simulink model "two"  (R2020b)
settings: Solver=VariableStepAuto  StartTime=0.0  StopTime=10.0  RelTol=1e-3
values from neighbouring files (symbols this model uses):
  be = 2.0    [variables.sldd]
  bv = 1.0    [variables.sldd]
  Ie = 1.0    [variables.sldd]
  Iv = 5.0    [variables.sldd]
  muk = 1.0    [variables.sldd]
  mus = 1.5    [variables.sldd]
  R = 1.0    [variables.sldd]
settings Model: Creator=USER  LastModifiedBy=USER

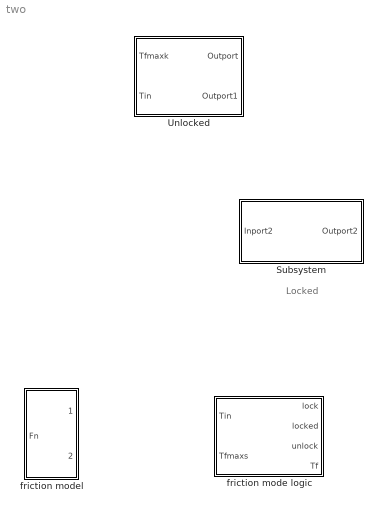
== system two ==
  note: Locked
  Subsystem : Subsystem
  Unlocked : Subsystem
  friction mode logic : Subsystem
  friction model : Subsystem

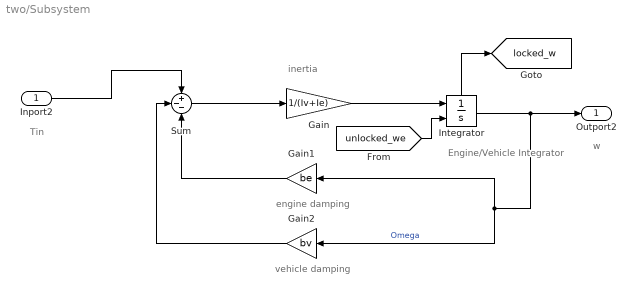
== system two/Subsystem ==
  note: w
  note: Tin
  note: inertia
  note: vehicle damping
  note: engine damping
  note: Engine/Vehicle
      | Integrator
  Inport2 : Inport
  Gain : Gain  Gain=1/(Iv+Ie)
  Gain1 : Gain  Gain=be
  Gain2 : Gain  Gain=bv
  Integrator : Integrator  InitialConditionSource=external  ShowStatePort=on
  Sum : Sum  Inputs=+--
  Outport2 : Outport
  tag scope: locked_w=global
  wires:
  [unlocked_we] -> Integrator/2
  Integrator/1 -> Outport2/1, Gain2/1, Gain1/1  "Omega"
  Gain/1 -> Integrator/1
  Integrator/State -> [locked_w]
  Sum/1 -> Gain/1
  Gain2/1 -> Sum/2
  Gain1/1 -> Sum/3
  Inport2/1 -> Sum/1

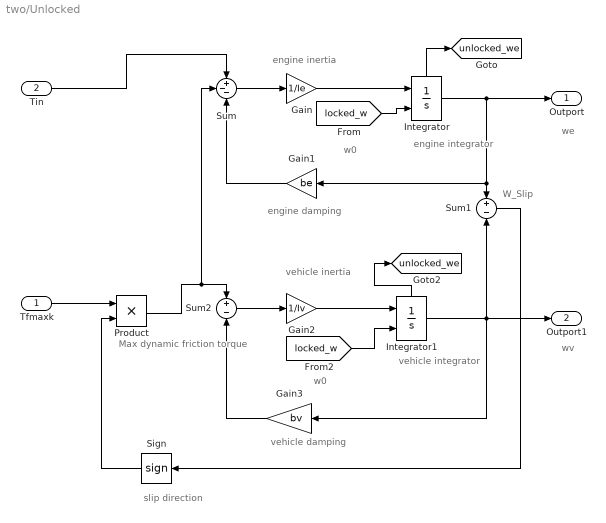
== system two/Unlocked ==
  note: we
  note: wv
  note: W_Slip
  note: vehicle
      | integrator
  note: engine
      | integrator
  note: w0
  note: w0
  note: engine damping
  note: engine inertia
  note: vehicle
      | inertia
  note: vehicle
      | damping
  note: slip direction
  note: Max
      | dynamic
      | friction
      | torque
  Tfmaxk : Inport
  Tin : Inport  Port=2
  Gain : Gain  Gain=1/Ie
  Gain1 : Gain  Gain=be
  Gain2 : Gain  Gain=1/Iv
  Gain3 : Gain  Gain=bv
  Integrator : Integrator  InitialConditionSource=external  ShowStatePort=on  ZeroCross=off
  Integrator1 : Integrator  InitialConditionSource=external  ShowStatePort=on  ZeroCross=off
  Product : Product
  Sign : Signum
  Sum : Sum  Inputs=+--
  Sum1 : Sum  Inputs=+-
  Sum2 : Sum  Inputs=+-
  Outport : Outport
  Outport1 : Outport  Port=2
  tag scope: unlocked_we=global
  wires:
  Sum/1 -> Gain/1
  Tfmaxk/1 -> Product/1
  Sum2/1 -> Gain2/1
  Sum1/1 -> Sign/1
  Integrator1/State -> [unlocked_we]
  Sign/1 -> Product/2
  Gain2/1 -> Integrator1/1
  Integrator/1 -> Outport/1, Gain1/1, Sum1/1
  [locked_w] -> Integrator1/2
  Integrator1/1 -> Outport1/1, Sum1/2, Gain3/1
  Product/1 -> Sum/2, Sum2/1
  Gain/1 -> Integrator/1
  Gain1/1 -> Sum/3
  Gain3/1 -> Sum2/2
  Tin/1 -> Sum/1
  [locked_w] -> Integrator/2
  Integrator/State -> [unlocked_we]

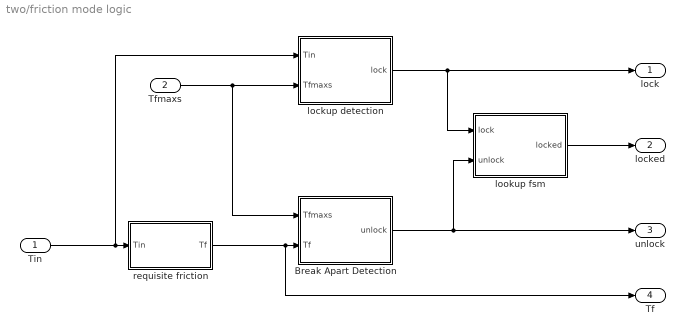
== system two/friction mode logic ==
  Tin : Inport
  Tfmaxs : Inport  Port=2
  Break Apart Detection : Subsystem
  lockup detection : Subsystem
  lookup fsm : Subsystem
  requisite friction : Subsystem
  lock : Outport
  locked : Outport  Port=2
  unlock : Outport  Port=3
  Tf : Outport  Port=4
  wires:
  Tfmaxs/1 -> Break Apart Detection/1(Tfmaxs), lockup detection/2(Tfmaxs)
  lockup detection/1(lock) -> lock/1, lookup fsm/1(lock)
  Break Apart Detection/1(unlock) -> unlock/1, lookup fsm/2(unlock)
  lookup fsm/1(locked) -> locked/1
  requisite friction/1(Tf) -> Tf/1, Break Apart Detection/2(Tf)
  Tin/1 -> lockup detection/1(Tin), requisite friction/1(Tin)

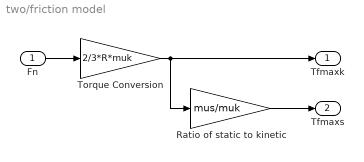
== system two/friction model ==
  Fn : Inport
  Ratio of static to kinetic : Gain  Gain=mus/muk  SaturateOnIntegerOverflow=on  OutDataTypeStr=Inherit: Same as input  ParamDataTypeStr=Inherit: Same as input
  Torque Conversion : Gain  Gain=2/3*R*muk  SaturateOnIntegerOverflow=on  OutDataTypeStr=Inherit: Same as input  ParamDataTypeStr=Inherit: Same as input
  Tfmaxk : Outport  InitialOutput=0  VectorParamsAs1DForOutWhenUnconnected=off
  Tfmaxs : Outport  Port=2  InitialOutput=0  VectorParamsAs1DForOutWhenUnconnected=off
  wires:
  Torque Conversion/1 -> Tfmaxk/1, Ratio of static to kinetic/1
  Fn/1 -> Torque Conversion/1
  Ratio of static to kinetic/1 -> Tfmaxs/1

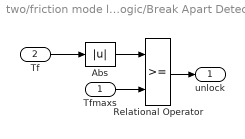
== system two/friction mode logic/Break Apart Detection ==
  Tfmaxs : Inport
  Tf : Inport  Port=2
  Abs : Abs  SaturateOnIntegerOverflow=on
  Relational Operator : RelationalOperator  OutDataTypeStr=boolean  RndMeth=Nearest  InputSameDT=on
  unlock : Outport  InitialOutput=0  VectorParamsAs1DForOutWhenUnconnected=off
  wires:
  Tf/1 -> Abs/1
  Relational Operator/1 -> unlock/1
  Abs/1 -> Relational Operator/1
  Tfmaxs/1 -> Relational Operator/2

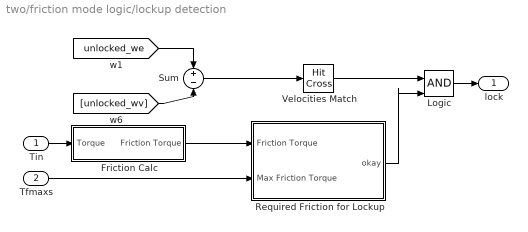
== system two/friction mode logic/lockup detection ==
  Tin : Inport
  Tfmaxs : Inport  Port=2
  Friction Calc : Subsystem
  Logic : Logic  IconShape=distinctive  OutDataTypeStr=boolean
  Required Friction for Lockup : Subsystem
  Sum : Sum  Inputs=+-  InputSameDT=on  SaturateOnIntegerOverflow=on  OutDataTypeStr=Inherit: Same as first input
  Velocities Match : HitCross
  lock : Outport  InitialOutput=0  VectorParamsAs1DForOutWhenUnconnected=off
  wires:
  Friction Calc/1(Friction Torque) -> Required Friction for Lockup/1(Friction Torque)
  Tfmaxs/1 -> Required Friction for Lockup/2(Max Friction Torque)
  Velocities Match/1 -> Logic/1
  Logic/1 -> lock/1
  Required Friction for Lockup/1(okay) -> Logic/2
  [unlocked_we] -> Sum/1
  [unlocked_wv] -> Sum/2
  Sum/1 -> Velocities Match/1
  Tin/1 -> Friction Calc/1(Torque)

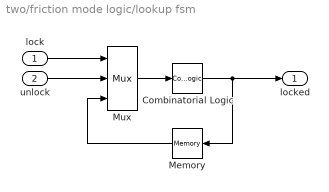
== system two/friction mode logic/lookup fsm ==
  lock : Inport
  unlock : Inport  Port=2
  Combinatorial Logic : CombinatorialLogic  TruthTable=[0;1;0;0;1;1;1;0]
  Memory : Memory
  Mux : Mux  Inputs=3
  locked : Outport  InitialOutput=0  VectorParamsAs1DForOutWhenUnconnected=off
  wires:
  Mux/1 -> Combinatorial Logic/1
  unlock/1 -> Mux/2
  Combinatorial Logic/1 -> locked/1, Memory/1
  lock/1 -> Mux/1
  Memory/1 -> Mux/3

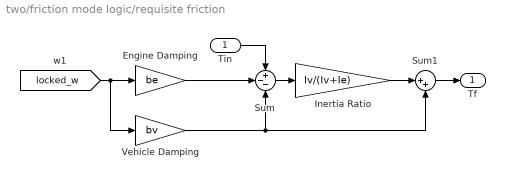
== system two/friction mode logic/requisite friction ==
  Tin : Inport
  Engine Damping : Gain  Gain=be  SaturateOnIntegerOverflow=on  OutDataTypeStr=Inherit: Same as input  ParamDataTypeStr=Inherit: Same as input
  Inertia Ratio : Gain  Gain=Iv/(Iv+Ie)  SaturateOnIntegerOverflow=on  OutDataTypeStr=Inherit: Same as input  ParamDataTypeStr=Inherit: Same as input
  Sum : Sum  Inputs=+--  InputSameDT=on  SaturateOnIntegerOverflow=on  OutDataTypeStr=Inherit: Same as first input
  Sum1 : Sum  Inputs=|++  InputSameDT=on  SaturateOnIntegerOverflow=on  OutDataTypeStr=Inherit: Same as first input
  Vehicle Damping : Gain  Gain=bv  SaturateOnIntegerOverflow=on  OutDataTypeStr=Inherit: Same as input  ParamDataTypeStr=Inherit: Same as input
  Tf : Outport  InitialOutput=0  VectorParamsAs1DForOutWhenUnconnected=off
  wires:
  [locked_w] -> Vehicle Damping/1, Engine Damping/1
  Engine Damping/1 -> Sum/2
  Vehicle Damping/1 -> Sum/3, Sum1/2
  Sum/1 -> Inertia Ratio/1
  Tin/1 -> Sum/1
  Inertia Ratio/1 -> Sum1/1
  Sum1/1 -> Tf/1

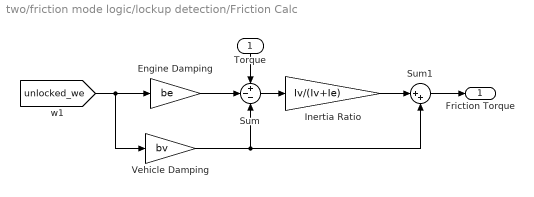
== system two/friction mode logic/lockup detection/Friction Calc ==
  Torque : Inport
  Engine Damping : Gain  Gain=be  SaturateOnIntegerOverflow=on  OutDataTypeStr=Inherit: Same as input  ParamDataTypeStr=Inherit: Same as input
  Inertia Ratio : Gain  Gain=Iv/(Iv+Ie)  SaturateOnIntegerOverflow=on  OutDataTypeStr=Inherit: Same as input  ParamDataTypeStr=Inherit: Same as input
  Sum : Sum  Inputs=+--  InputSameDT=on  SaturateOnIntegerOverflow=on  OutDataTypeStr=Inherit: Same as first input
  Sum1 : Sum  Inputs=|++  InputSameDT=on  SaturateOnIntegerOverflow=on  OutDataTypeStr=Inherit: Same as first input
  Vehicle Damping : Gain  Gain=bv  SaturateOnIntegerOverflow=on  OutDataTypeStr=Inherit: Same as input  ParamDataTypeStr=Inherit: Same as input
  Friction Torque : Outport  InitialOutput=0  VectorParamsAs1DForOutWhenUnconnected=off
  wires:
  [unlocked_we] -> Engine Damping/1, Vehicle Damping/1
  Vehicle Damping/1 -> Sum1/2, Sum/3
  Engine Damping/1 -> Sum/2
  Sum/1 -> Inertia Ratio/1
  Torque/1 -> Sum/1
  Inertia Ratio/1 -> Sum1/1
  Sum1/1 -> Friction Torque/1

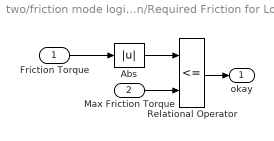
== system two/friction mode logic/lockup detection/Required Friction for Lockup ==
  Friction Torque : Inport
  Max Friction Torque : Inport  Port=2
  Abs : Abs  SaturateOnIntegerOverflow=on
  Relational Operator : RelationalOperator  Operator=<=  OutDataTypeStr=boolean  RndMeth=Nearest  InputSameDT=on
  okay : Outport  InitialOutput=0  VectorParamsAs1DForOutWhenUnconnected=off
  wires:
  Friction Torque/1 -> Abs/1
  Relational Operator/1 -> okay/1
  Abs/1 -> Relational Operator/1
  Max Friction Torque/1 -> Relational Operator/2
